simulink model "VIPRExit557TrgtPos"  (R2018b)
settings: Solver=FixedStepDiscrete  StartTime=0.0  StopTime=10.0  RelTol=1e-3
undefined symbols (not defined in the file or in its folder): arg, Rte_EEP_VIPRExitPassStBkReclnTrgtPos_Set, Rte_EEP_VIPRExitPassStFwdBkwdTrgtPos_Set, Rte_EEP_VIPRExitSecRwRtStBkReclnTrgtPos_Set, Rte_EEP_VIPRExitSecRwRtStCushFrntTrgtPos_Set, Rte_EEP_VIPRExitSecRwRtStFwdBkwdTrgtPos_Set, Rte_EEP_VIPRExitSecRwRtStLgrstInwdOtwdTrgtPos_Set, Rte_EEP_VIPRExitSecRwRtStLgrstUpwdDnwdTrgtPos_Set, Rte_EEP_VIPRExitThdRwLtStBkReclnTrgtPos_Set, Rte_EEP_VIPRExitThdRwLtStFwdBkwdTrgtPos_Set, Rte_EEP_VIPRExitThdRwRtStBkReclnTrgtPos_Set, Rte_EEP_VIPRExitThdRwRtStFwdBkwdTrgtPos_Set
settings Model: ModifiedHistory=2024.7.10 V3.0.0 557模式流程V1.9  Creator=sn2xws  LastModifiedBy=sn2xws
settings DataIOCC: SaveFormat=StructureWithTime
settings OptimizationCC: DefaultParameterBehavior=Inlined  EnhancedBackFolding=on  PassReuseOutputArgsAs=Individual arguments  ZeroExternalMemoryAtStartup=off  ZeroInternalMemoryAtStartup=off  OptimizeBlockOrder=speed  DifferentSizesBufferReuse=on  OptimizationCustomize=off
settings DebuggingCC: ParameterTunabilityLossMsg=error
settings SFSimCC: MATLABDynamicMemAlloc=off
settings RTWCC: SystemTargetFile=autosar.tlc  GenCodeOnly=on  TemplateMakefile=ert_default_tmf  Description=AUTOSAR  GenerateReport=on  IncludeHyperlinkInReport=on  LaunchReport=on  GenerateTraceInfo=on  GenerateTraceReport=on  GenerateTraceReportSl=on  GenerateTraceReportSf=on  GenerateTraceReportEml=on
settings CodeAppCC: ForceParamTrailComments=on  IgnoreCustomStorageClasses=off  OperatorAnnotations=on  SimulinkDataObjDesc=on  SFDataObjDesc=on  InsertBlockDesc=on
settings STFCustomTargetCC: TargetLangStandard=C99 (ISO)  MultiwordLength=256  ParMdlRefBuildCompliant=on  CompOptLevelCompliant=on  IncludeMdlTerminateFcn=off  CombineOutputUpdateFcns=on  SuppressErrorStatus=on  ERTCustomFileBanners=on  SupportNonFinite=off  SupportComplex=off  SupportContinuousTime=off  SupportNonInlinedSFcns=off  RemoveResetFunc=on  MATLABClassNameForMDSCustomization=Simulink.SoftwareTarget.ERTCustomization  AutosarCompliant=on  UseToolchainInfoCompliant=on  LookupTableObjectStructAxisOrder=2,1,3,4,...  LUTObjectStructOrderEvenSpacing=Size,Table,Breakpoints  SystemTargetFile=autosar.tlc
settings ERTTargetCC: TargetLangStandard=C99 (ISO)  ConcurrentExecutionCompliant=off  IncludeMdlTerminateFcn=off  SuppressErrorStatus=on  SupportNonFinite=off  SupportComplex=off  ModelStepFunctionPrototypeControlCompliant=off  CPPClassGenCompliant=off  AutosarCompliant=on  LookupTableObjectStructAxisOrder=2,1,3,4,...  LUTObjectStructOrderEvenSpacing=Size,Table,Breakpoints  InlinedParameterPlacement=NonHierarchical  ERTCustomFileTemplate=example_file_process.tlc  ERTFilePackagingFormat=Compact

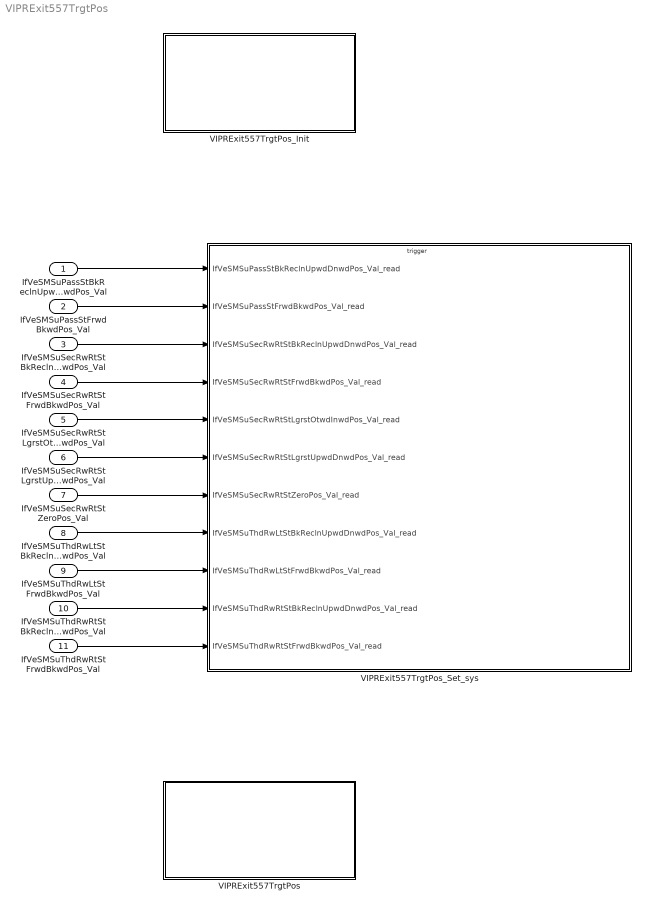
== system VIPRExit557TrgtPos ==
  IfVeSMSuPassStBkReclnUpwdDnwdPos_Val : Inport  OutDataTypeStr=uint16  PortDimensions=1
  IfVeSMSuPassStFrwdBkwdPos_Val : Inport  Port=2  OutDataTypeStr=uint16  PortDimensions=1
  IfVeSMSuSecRwRtStBkReclnUpwdDnwdPos_Val : Inport  Port=3  OutDataTypeStr=uint16  PortDimensions=1
  IfVeSMSuSecRwRtStFrwdBkwdPos_Val : Inport  Port=4  OutDataTypeStr=uint16  PortDimensions=1
  IfVeSMSuSecRwRtStLgrstOtwdInwdPos_Val : Inport  Port=5  OutDataTypeStr=uint16  PortDimensions=1
  IfVeSMSuSecRwRtStLgrstUpwdDnwdPos_Val : Inport  Port=6  OutDataTypeStr=uint16  PortDimensions=1
  IfVeSMSuSecRwRtStZeroPos_Val : Inport  Port=7  OutDataTypeStr=uint16  PortDimensions=1
  IfVeSMSuThdRwLtStBkReclnUpwdDnwdPos_Val : Inport  Port=8  OutDataTypeStr=uint16  PortDimensions=1
  IfVeSMSuThdRwLtStFrwdBkwdPos_Val : Inport  Port=9  OutDataTypeStr=uint16  PortDimensions=1
  IfVeSMSuThdRwRtStBkReclnUpwdDnwdPos_Val : Inport  Port=10  OutDataTypeStr=uint16  PortDimensions=1
  IfVeSMSuThdRwRtStFrwdBkwdPos_Val : Inport  Port=11  OutDataTypeStr=uint16  PortDimensions=1
  VIPRExit557TrgtPos : Subsystem
  VIPRExit557TrgtPos_Init : Subsystem
  VIPRExit557TrgtPos_Set_sys : Subsystem
  wires:
  IfVeSMSuPassStBkReclnUpwdDnwdPos_Val/1 -> VIPRExit557TrgtPos_Set_sys/1(IfVeSMSuPassStBkReclnUpwdDnwdPos_Val_read)
  IfVeSMSuPassStFrwdBkwdPos_Val/1 -> VIPRExit557TrgtPos_Set_sys/2(IfVeSMSuPassStFrwdBkwdPos_Val_read)
  IfVeSMSuSecRwRtStBkReclnUpwdDnwdPos_Val/1 -> VIPRExit557TrgtPos_Set_sys/3(IfVeSMSuSecRwRtStBkReclnUpwdDnwdPos_Val_read)
  IfVeSMSuSecRwRtStFrwdBkwdPos_Val/1 -> VIPRExit557TrgtPos_Set_sys/4(IfVeSMSuSecRwRtStFrwdBkwdPos_Val_read)
  IfVeSMSuSecRwRtStLgrstOtwdInwdPos_Val/1 -> VIPRExit557TrgtPos_Set_sys/5(IfVeSMSuSecRwRtStLgrstOtwdInwdPos_Val_read)
  IfVeSMSuSecRwRtStLgrstUpwdDnwdPos_Val/1 -> VIPRExit557TrgtPos_Set_sys/6(IfVeSMSuSecRwRtStLgrstUpwdDnwdPos_Val_read)
  IfVeSMSuSecRwRtStZeroPos_Val/1 -> VIPRExit557TrgtPos_Set_sys/7(IfVeSMSuSecRwRtStZeroPos_Val_read)
  IfVeSMSuThdRwLtStBkReclnUpwdDnwdPos_Val/1 -> VIPRExit557TrgtPos_Set_sys/8(IfVeSMSuThdRwLtStBkReclnUpwdDnwdPos_Val_read)
  IfVeSMSuThdRwLtStFrwdBkwdPos_Val/1 -> VIPRExit557TrgtPos_Set_sys/9(IfVeSMSuThdRwLtStFrwdBkwdPos_Val_read)
  IfVeSMSuThdRwRtStBkReclnUpwdDnwdPos_Val/1 -> VIPRExit557TrgtPos_Set_sys/10(IfVeSMSuThdRwRtStBkReclnUpwdDnwdPos_Val_read)
  IfVeSMSuThdRwRtStFrwdBkwdPos_Val/1 -> VIPRExit557TrgtPos_Set_sys/11(IfVeSMSuThdRwRtStFrwdBkwdPos_Val_read)

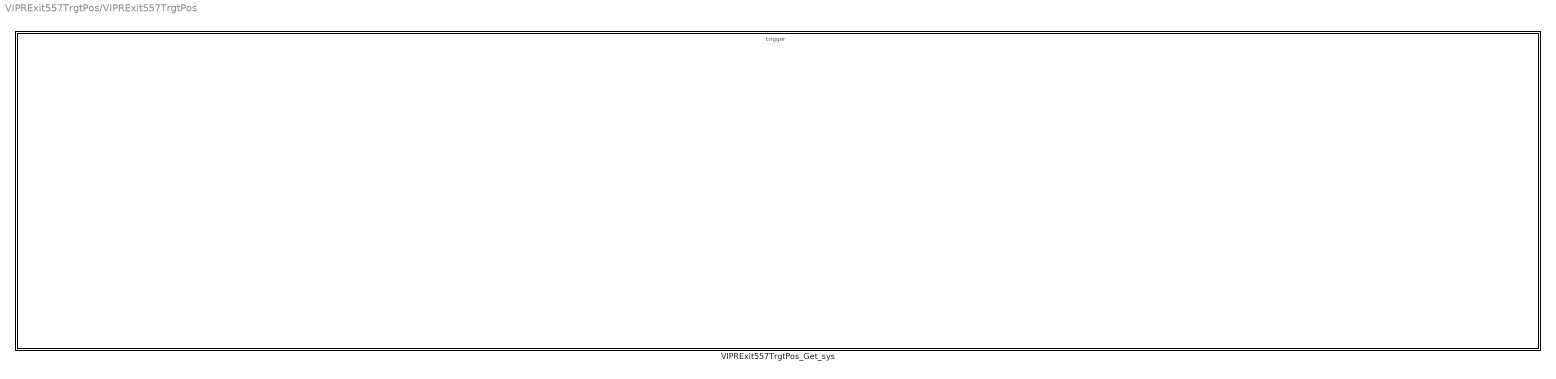
== system VIPRExit557TrgtPos/VIPRExit557TrgtPos ==
  VIPRExit557TrgtPos_Get_sys : Subsystem

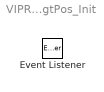
== system VIPRExit557TrgtPos/VIPRExit557TrgtPos_Init ==
  Event Listener : EventListener  EventName=reset

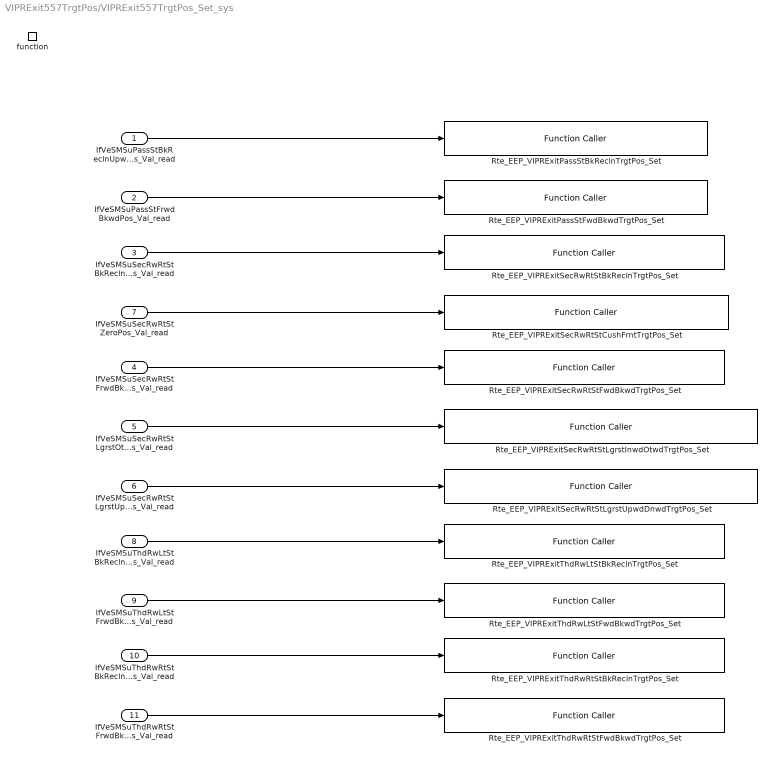
== system VIPRExit557TrgtPos/VIPRExit557TrgtPos_Set_sys ==
  IfVeSMSuPassStBkReclnUpwdDnwdPos_Val_read : Inport
  IfVeSMSuPassStFrwdBkwdPos_Val_read : Inport  Port=2
  IfVeSMSuSecRwRtStBkReclnUpwdDnwdPos_Val_read : Inport  Port=3
  IfVeSMSuSecRwRtStFrwdBkwdPos_Val_read : Inport  Port=4
  IfVeSMSuSecRwRtStLgrstOtwdInwdPos_Val_read : Inport  Port=5
  IfVeSMSuSecRwRtStLgrstUpwdDnwdPos_Val_read : Inport  Port=6
  IfVeSMSuSecRwRtStZeroPos_Val_read : Inport  Port=7
  IfVeSMSuThdRwLtStBkReclnUpwdDnwdPos_Val_read : Inport  Port=8
  IfVeSMSuThdRwLtStFrwdBkwdPos_Val_read : Inport  Port=9
  IfVeSMSuThdRwRtStBkReclnUpwdDnwdPos_Val_read : Inport  Port=10
  IfVeSMSuThdRwRtStFrwdBkwdPos_Val_read : Inport  Port=11
  function : TriggerPort  TriggerType=function-call  IsSimulinkFunction=on  FunctionName=VIPRExit557TrgtPos_Set  VariantControl=(inherit)
  Rte_EEP_VIPRExitPassStBkReclnTrgtPos_Set : FunctionCaller  FunctionPrototype=Rte_EEP_VIPRExitPassStBkReclnTrgtPos_Set(arg)  InputArgumentSpecifications=P_EEP_Uint16
  Rte_EEP_VIPRExitPassStFwdBkwdTrgtPos_Set : FunctionCaller  FunctionPrototype=Rte_EEP_VIPRExitPassStFwdBkwdTrgtPos_Set(arg)  InputArgumentSpecifications=P_EEP_Uint16
  Rte_EEP_VIPRExitSecRwRtStBkReclnTrgtPos_Set : FunctionCaller  FunctionPrototype=Rte_EEP_VIPRExitSecRwRtStBkReclnTrgtPos_Set(arg)  InputArgumentSpecifications=P_EEP_Uint16
  Rte_EEP_VIPRExitSecRwRtStCushFrntTrgtPos_Set : FunctionCaller  FunctionPrototype=Rte_EEP_VIPRExitSecRwRtStCushFrntTrgtPos_Set(arg)  InputArgumentSpecifications=P_EEP_Uint16
  Rte_EEP_VIPRExitSecRwRtStFwdBkwdTrgtPos_Set : FunctionCaller  FunctionPrototype=Rte_EEP_VIPRExitSecRwRtStFwdBkwdTrgtPos_Set(arg)  InputArgumentSpecifications=P_EEP_Uint16
  Rte_EEP_VIPRExitSecRwRtStLgrstInwdOtwdTrgtPos_Set : FunctionCaller  FunctionPrototype=Rte_EEP_VIPRExitSecRwRtStLgrstInwdOtwdTrgtPos_Set(arg)  InputArgumentSpecifications=P_EEP_Uint16
  Rte_EEP_VIPRExitSecRwRtStLgrstUpwdDnwdTrgtPos_Set : FunctionCaller  FunctionPrototype=Rte_EEP_VIPRExitSecRwRtStLgrstUpwdDnwdTrgtPos_Set(arg)  InputArgumentSpecifications=P_EEP_Uint16
  Rte_EEP_VIPRExitThdRwLtStBkReclnTrgtPos_Set : FunctionCaller  FunctionPrototype=Rte_EEP_VIPRExitThdRwLtStBkReclnTrgtPos_Set(arg)  InputArgumentSpecifications=P_EEP_Uint16
  Rte_EEP_VIPRExitThdRwLtStFwdBkwdTrgtPos_Set : FunctionCaller  FunctionPrototype=Rte_EEP_VIPRExitThdRwLtStFwdBkwdTrgtPos_Set(arg)  InputArgumentSpecifications=P_EEP_Uint16
  Rte_EEP_VIPRExitThdRwRtStBkReclnTrgtPos_Set : FunctionCaller  FunctionPrototype=Rte_EEP_VIPRExitThdRwRtStBkReclnTrgtPos_Set(arg)  InputArgumentSpecifications=P_EEP_Uint16
  Rte_EEP_VIPRExitThdRwRtStFwdBkwdTrgtPos_Set : FunctionCaller  FunctionPrototype=Rte_EEP_VIPRExitThdRwRtStFwdBkwdTrgtPos_Set(arg)  InputArgumentSpecifications=P_EEP_Uint16
  wires:
  IfVeSMSuPassStBkReclnUpwdDnwdPos_Val_read/1 -> Rte_EEP_VIPRExitPassStBkReclnTrgtPos_Set/1
  IfVeSMSuPassStFrwdBkwdPos_Val_read/1 -> Rte_EEP_VIPRExitPassStFwdBkwdTrgtPos_Set/1
  IfVeSMSuSecRwRtStBkReclnUpwdDnwdPos_Val_read/1 -> Rte_EEP_VIPRExitSecRwRtStBkReclnTrgtPos_Set/1
  IfVeSMSuSecRwRtStZeroPos_Val_read/1 -> Rte_EEP_VIPRExitSecRwRtStCushFrntTrgtPos_Set/1
  IfVeSMSuSecRwRtStFrwdBkwdPos_Val_read/1 -> Rte_EEP_VIPRExitSecRwRtStFwdBkwdTrgtPos_Set/1
  IfVeSMSuSecRwRtStLgrstOtwdInwdPos_Val_read/1 -> Rte_EEP_VIPRExitSecRwRtStLgrstInwdOtwdTrgtPos_Set/1
  IfVeSMSuSecRwRtStLgrstUpwdDnwdPos_Val_read/1 -> Rte_EEP_VIPRExitSecRwRtStLgrstUpwdDnwdTrgtPos_Set/1
  IfVeSMSuThdRwLtStBkReclnUpwdDnwdPos_Val_read/1 -> Rte_EEP_VIPRExitThdRwLtStBkReclnTrgtPos_Set/1
  IfVeSMSuThdRwLtStFrwdBkwdPos_Val_read/1 -> Rte_EEP_VIPRExitThdRwLtStFwdBkwdTrgtPos_Set/1
  IfVeSMSuThdRwRtStBkReclnUpwdDnwdPos_Val_read/1 -> Rte_EEP_VIPRExitThdRwRtStBkReclnTrgtPos_Set/1
  IfVeSMSuThdRwRtStFrwdBkwdPos_Val_read/1 -> Rte_EEP_VIPRExitThdRwRtStFwdBkwdTrgtPos_Set/1

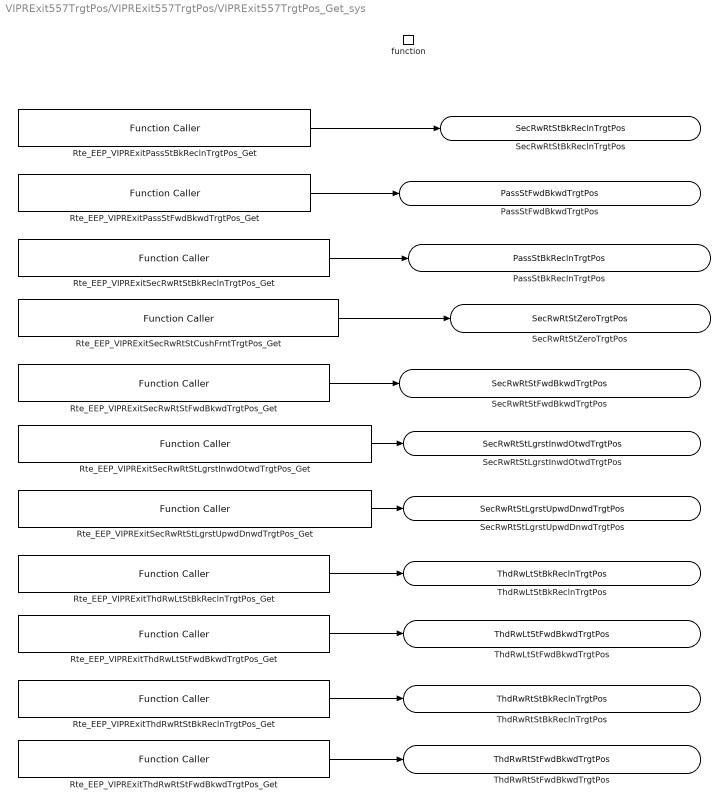
== system VIPRExit557TrgtPos/VIPRExit557TrgtPos/VIPRExit557TrgtPos_Get_sys ==
  function : TriggerPort  TriggerType=function-call  IsSimulinkFunction=on  FunctionName=VIPRExit557TrgtPos_Get  VariantControl=(inherit)
  Rte_EEP_VIPRExitPassStBkReclnTrgtPos_Get : FunctionCaller  FunctionPrototype=arg = Rte_EEP_VIPRExitPassStBkReclnTrgtPos_Get()  OutputArgumentSpecifications=P_EEP_Uint16
  Rte_EEP_VIPRExitPassStFwdBkwdTrgtPos_Get : FunctionCaller  FunctionPrototype=arg = Rte_EEP_VIPRExitPassStFwdBkwdTrgtPos_Get()  OutputArgumentSpecifications=P_EEP_Uint16
  Rte_EEP_VIPRExitSecRwRtStBkReclnTrgtPos_Get : FunctionCaller  FunctionPrototype=arg = Rte_EEP_VIPRExitSecRwRtStBkReclnTrgtPos_Get()  OutputArgumentSpecifications=P_EEP_Uint16
  Rte_EEP_VIPRExitSecRwRtStCushFrntTrgtPos_Get : FunctionCaller  FunctionPrototype=arg = Rte_EEP_VIPRExitSecRwRtStCushFrntTrgtPos_Get()  OutputArgumentSpecifications=P_EEP_Uint16
  Rte_EEP_VIPRExitSecRwRtStFwdBkwdTrgtPos_Get : FunctionCaller  FunctionPrototype=arg = Rte_EEP_VIPRExitSecRwRtStFwdBkwdTrgtPos_Get()  OutputArgumentSpecifications=P_EEP_Uint16
  Rte_EEP_VIPRExitSecRwRtStLgrstInwdOtwdTrgtPos_Get : FunctionCaller  FunctionPrototype=arg = Rte_EEP_VIPRExitSecRwRtStLgrstInwdOtwdTrgtPos_Get()  OutputArgumentSpecifications=P_EEP_Uint16
  Rte_EEP_VIPRExitSecRwRtStLgrstUpwdDnwdTrgtPos_Get : FunctionCaller  FunctionPrototype=arg = Rte_EEP_VIPRExitSecRwRtStLgrstUpwdDnwdTrgtPos_Get()  OutputArgumentSpecifications=P_EEP_Uint16
  Rte_EEP_VIPRExitThdRwLtStBkReclnTrgtPos_Get : FunctionCaller  FunctionPrototype=arg = Rte_EEP_VIPRExitThdRwLtStBkReclnTrgtPos_Get()  OutputArgumentSpecifications=P_EEP_Uint16
  Rte_EEP_VIPRExitThdRwLtStFwdBkwdTrgtPos_Get : FunctionCaller  FunctionPrototype=arg = Rte_EEP_VIPRExitThdRwLtStFwdBkwdTrgtPos_Get()  OutputArgumentSpecifications=P_EEP_Uint16
  Rte_EEP_VIPRExitThdRwRtStBkReclnTrgtPos_Get : FunctionCaller  FunctionPrototype=arg = Rte_EEP_VIPRExitThdRwRtStBkReclnTrgtPos_Get()  OutputArgumentSpecifications=P_EEP_Uint16
  Rte_EEP_VIPRExitThdRwRtStFwdBkwdTrgtPos_Get : FunctionCaller  FunctionPrototype=arg = Rte_EEP_VIPRExitThdRwRtStFwdBkwdTrgtPos_Get()  OutputArgumentSpecifications=P_EEP_Uint16
  SecRwRtStBkReclnTrgtPos : ArgOut  OutDataTypeStr=uint16  ArgumentName=SecRwRtStBkReclnTrgtPos
  SecRwRtStZeroTrgtPos : ArgOut  Port=2  OutDataTypeStr=uint16  ArgumentName=SecRwRtStZeroTrgtPos
  SecRwRtStLgrstUpwdDnwdTrgtPos : ArgOut  Port=3  OutDataTypeStr=uint16  ArgumentName=SecRwRtStLgrstUpwdDnwdTrgtPos
  SecRwRtStLgrstInwdOtwdTrgtPos : ArgOut  Port=4  OutDataTypeStr=uint16  ArgumentName=SecRwRtStLgrstInwdOtwdTrgtPos
  ThdRwLtStBkReclnTrgtPos : ArgOut  Port=5  OutDataTypeStr=uint16  ArgumentName=ThdRwLtStBkReclnTrgtPos
  ThdRwLtStFwdBkwdTrgtPos : ArgOut  Port=6  OutDataTypeStr=uint16  ArgumentName=ThdRwLtStFwdBkwdTrgtPos
  ThdRwRtStBkReclnTrgtPos : ArgOut  Port=7  OutDataTypeStr=uint16  ArgumentName=ThdRwRtStBkReclnTrgtPos
  ThdRwRtStFwdBkwdTrgtPos : ArgOut  Port=8  OutDataTypeStr=uint16  ArgumentName=ThdRwRtStFwdBkwdTrgtPos
  PassStBkReclnTrgtPos : ArgOut  Port=9  OutDataTypeStr=uint16  ArgumentName=PassStBkReclnTrgtPos
  PassStFwdBkwdTrgtPos : ArgOut  Port=10  OutDataTypeStr=uint16  ArgumentName=PassStFwdBkwdTrgtPos
  SecRwRtStFwdBkwdTrgtPos : ArgOut  Port=11  OutDataTypeStr=uint16  ArgumentName=SecRwRtStFwdBkwdTrgtPos
  wires:
  Rte_EEP_VIPRExitPassStBkReclnTrgtPos_Get/1 -> SecRwRtStBkReclnTrgtPos/1
  Rte_EEP_VIPRExitPassStFwdBkwdTrgtPos_Get/1 -> PassStFwdBkwdTrgtPos/1
  Rte_EEP_VIPRExitSecRwRtStBkReclnTrgtPos_Get/1 -> PassStBkReclnTrgtPos/1
  Rte_EEP_VIPRExitSecRwRtStCushFrntTrgtPos_Get/1 -> SecRwRtStZeroTrgtPos/1
  Rte_EEP_VIPRExitSecRwRtStFwdBkwdTrgtPos_Get/1 -> SecRwRtStFwdBkwdTrgtPos/1
  Rte_EEP_VIPRExitSecRwRtStLgrstInwdOtwdTrgtPos_Get/1 -> SecRwRtStLgrstInwdOtwdTrgtPos/1
  Rte_EEP_VIPRExitSecRwRtStLgrstUpwdDnwdTrgtPos_Get/1 -> SecRwRtStLgrstUpwdDnwdTrgtPos/1
  Rte_EEP_VIPRExitThdRwLtStBkReclnTrgtPos_Get/1 -> ThdRwLtStBkReclnTrgtPos/1
  Rte_EEP_VIPRExitThdRwLtStFwdBkwdTrgtPos_Get/1 -> ThdRwLtStFwdBkwdTrgtPos/1
  Rte_EEP_VIPRExitThdRwRtStBkReclnTrgtPos_Get/1 -> ThdRwRtStBkReclnTrgtPos/1
  Rte_EEP_VIPRExitThdRwRtStFwdBkwdTrgtPos_Get/1 -> ThdRwRtStFwdBkwdTrgtPos/1
